simulink model "ASDrf_SelectParameter"  (R2016b)
settings: configuration reference "CodeGenConfigSet" (kept outside this file)
values from neighbouring files (symbols this model uses):
  ASDrf_facGovNegGear0_CUR = Calibration.Parameter    [init_ASDrf_SelectParameter.m]    (also in init_ASDrf_SelectParameter_SIL.m = Simulink.Parameter)
  ASDrf_facGovNegGear0_CURX = Calibration.Parameter    [init_ASDrf_SelectParameter.m]    (also in init_ASDrf_SelectParameter_SIL.m = Simulink.Parameter)
  ASDrf_facGovNegGear1_CUR = Calibration.Parameter    [init_ASDrf_SelectParameter.m]    (also in init_ASDrf_SelectParameter_SIL.m = Simulink.Parameter)
  ASDrf_facGovNegGear1_CURX = Calibration.Parameter    [init_ASDrf_SelectParameter.m]    (also in init_ASDrf_SelectParameter_SIL.m = Simulink.Parameter)
  ASDrf_facGovNegGear2_CUR = Calibration.Parameter    [init_ASDrf_SelectParameter.m]    (also in init_ASDrf_SelectParameter_SIL.m = Simulink.Parameter)
  ASDrf_facGovNegGear2_CURX = Calibration.Parameter    [init_ASDrf_SelectParameter.m]    (also in init_ASDrf_SelectParameter_SIL.m = Simulink.Parameter)
  ASDrf_facGovNegGear3_CUR = Calibration.Parameter    [init_ASDrf_SelectParameter.m]    (also in init_ASDrf_SelectParameter_SIL.m = Simulink.Parameter)
  ASDrf_facGovNegGear3_CURX = Calibration.Parameter    [init_ASDrf_SelectParameter.m]    (also in init_ASDrf_SelectParameter_SIL.m = Simulink.Parameter)
  ASDrf_facGovNegGear4_CUR = Calibration.Parameter    [init_ASDrf_SelectParameter.m]    (also in init_ASDrf_SelectParameter_SIL.m = Simulink.Parameter)
  ASDrf_facGovNegGear4_CURX = Calibration.Parameter    [init_ASDrf_SelectParameter.m]    (also in init_ASDrf_SelectParameter_SIL.m = Simulink.Parameter)
  ASDrf_facGovNegGear5_CUR = Calibration.Parameter    [init_ASDrf_SelectParameter.m]    (also in init_ASDrf_SelectParameter_SIL.m = Simulink.Parameter)
  ASDrf_facGovNegGear5_CURX = Calibration.Parameter    [init_ASDrf_SelectParameter.m]    (also in init_ASDrf_SelectParameter_SIL.m = Simulink.Parameter)
  ASDrf_facGovPosGear0_CUR = Calibration.Parameter    [init_ASDrf_SelectParameter.m]    (also in init_ASDrf_SelectParameter_SIL.m = Simulink.Parameter)
  ASDrf_facGovPosGear0_CURX = Calibration.Parameter    [init_ASDrf_SelectParameter.m]    (also in init_ASDrf_SelectParameter_SIL.m = Simulink.Parameter)
  ASDrf_facGovPosGear1_CUR = Calibration.Parameter    [init_ASDrf_SelectParameter.m]    (also in init_ASDrf_SelectParameter_SIL.m = Simulink.Parameter)
  ASDrf_facGovPosGear1_CURX = Calibration.Parameter    [init_ASDrf_SelectParameter.m]    (also in init_ASDrf_SelectParameter_SIL.m = Simulink.Parameter)
  ASDrf_facGovPosGear2_CUR = Calibration.Parameter    [init_ASDrf_SelectParameter.m]    (also in init_ASDrf_SelectParameter_SIL.m = Simulink.Parameter)
  ASDrf_facGovPosGear2_CURX = Calibration.Parameter    [init_ASDrf_SelectParameter.m]    (also in init_ASDrf_SelectParameter_SIL.m = Simulink.Parameter)
  ASDrf_facGovPosGear3_CUR = Calibration.Parameter    [init_ASDrf_SelectParameter.m]    (also in init_ASDrf_SelectParameter_SIL.m = Simulink.Parameter)
  ASDrf_facGovPosGear3_CURX = Calibration.Parameter    [init_ASDrf_SelectParameter.m]    (also in init_ASDrf_SelectParameter_SIL.m = Simulink.Parameter)
  ASDrf_facGovPosGear4_CUR = Calibration.Parameter    [init_ASDrf_SelectParameter.m]    (also in init_ASDrf_SelectParameter_SIL.m = Simulink.Parameter)
  ASDrf_facGovPosGear4_CURX = Calibration.Parameter    [init_ASDrf_SelectParameter.m]    (also in init_ASDrf_SelectParameter_SIL.m = Simulink.Parameter)
  ASDrf_facGovPosGear5_CUR = Calibration.Parameter    [init_ASDrf_SelectParameter.m]    (also in init_ASDrf_SelectParameter_SIL.m = Simulink.Parameter)
  ASDrf_facGovPosGear5_CURX = Calibration.Parameter    [init_ASDrf_SelectParameter.m]    (also in init_ASDrf_SelectParameter_SIL.m = Simulink.Parameter)
undefined symbols (not defined in the file or in its folder): CEngDsT_tTransf_CURX
settings Model: Creator=lenovo  LastModifiedBy=wangrui
settings ConfigSetRef: SourceLocation=Base Workspace

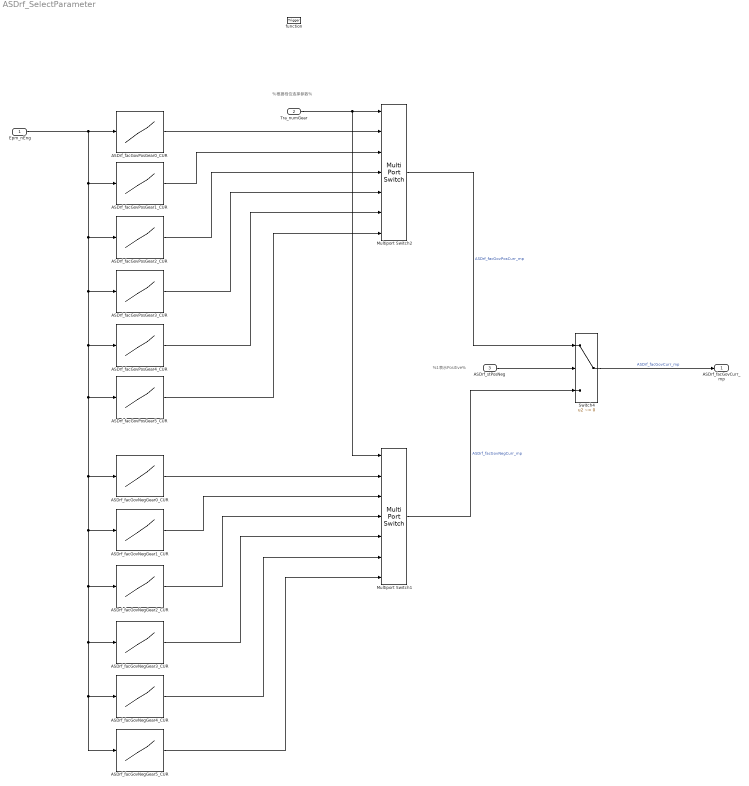
== system ASDrf_SelectParameter ==
  note: %根据档位选择参数%
  note: %1表示Positive%
  Epm_nEng : Inport  Tag=rpm  Description=Engine speed  OutMin=0  OutMax=6000  OutDataTypeStr=EngSpeed_rpm
  Tra_numGear : Inport  Description=Current gear information  Port=2  OutMin=-128  OutMax=127  OutDataTypeStr=Tra_num
  ASDrf_stPosNeg : Inport  Description=Positive or negative intervention status  Port=3  OutMin=0  OutMax=1  OutDataTypeStr=boolean
  function : TriggerPort  TriggerType=function-call  VariantControl=Variant
  ASDrf_facGovNegGear0_CUR : Lookup_n-D  RequirementInfo={} %GIDa_dec7f9a6_086f_4cd9_b948_1532d9a6f0c6  DialogController=Simulink.DDGSource  NumberOfTableDimensions=1  BreakpointsForDimension1=ASDrf_facGovNegGear0_CURX  BreakpointsForDimension2=CEngDsT_tTransf_CURX  IndexSearchMethod=Linear search  BeginIndexSearchUsingPreviousIndexResult=on  Table=ASDrf_facGovNegGear0_CUR  ExtrapMethod=Clip  UseLastTableValue=on  InternalRulePriority=Speed  OutDataTypeStr=Inherit: Inherit via back propagation  SaturateOnIntegerOverflow=on
  ASDrf_facGovNegGear1_CUR : Lookup_n-D  RequirementInfo={} %GIDa_8af62142_568a_4d65_a569_7be54cadb9a5  DialogController=Simulink.DDGSource  NumberOfTableDimensions=1  BreakpointsForDimension1=ASDrf_facGovNegGear1_CURX  BreakpointsForDimension2=CEngDsT_tTransf_CURX  IndexSearchMethod=Linear search  BeginIndexSearchUsingPreviousIndexResult=on  Table=ASDrf_facGovNegGear1_CUR  ExtrapMethod=Clip  UseLastTableValue=on  InternalRulePriority=Speed  OutDataTypeStr=Inherit: Inherit via back propagation  SaturateOnIntegerOverflow=on
  ASDrf_facGovNegGear2_CUR : Lookup_n-D  RequirementInfo={} %GIDa_3d8b842d_bc8c_4451_b7a4_3a6bb0e5109c  DialogController=Simulink.DDGSource  NumberOfTableDimensions=1  BreakpointsForDimension1=ASDrf_facGovNegGear2_CURX  BreakpointsForDimension2=CEngDsT_tTransf_CURX  IndexSearchMethod=Linear search  BeginIndexSearchUsingPreviousIndexResult=on  Table=ASDrf_facGovNegGear2_CUR  ExtrapMethod=Clip  UseLastTableValue=on  InternalRulePriority=Speed  OutDataTypeStr=Inherit: Inherit via back propagation  SaturateOnIntegerOverflow=on
  ASDrf_facGovNegGear3_CUR : Lookup_n-D  RequirementInfo={} %GIDa_717010b1_d4d2_4a42_82df_177817b4661e  DialogController=Simulink.DDGSource  NumberOfTableDimensions=1  BreakpointsForDimension1=ASDrf_facGovNegGear3_CURX  BreakpointsForDimension2=CEngDsT_tTransf_CURX  IndexSearchMethod=Linear search  BeginIndexSearchUsingPreviousIndexResult=on  Table=ASDrf_facGovNegGear3_CUR  ExtrapMethod=Clip  UseLastTableValue=on  InternalRulePriority=Speed  OutDataTypeStr=Inherit: Inherit via back propagation  SaturateOnIntegerOverflow=on
  ASDrf_facGovNegGear4_CUR : Lookup_n-D  RequirementInfo={} %GIDa_d036bcad_9456_44a3_9c9b_0a91d5bad276  DialogController=Simulink.DDGSource  NumberOfTableDimensions=1  BreakpointsForDimension1=ASDrf_facGovNegGear4_CURX  BreakpointsForDimension2=CEngDsT_tTransf_CURX  IndexSearchMethod=Linear search  BeginIndexSearchUsingPreviousIndexResult=on  Table=ASDrf_facGovNegGear4_CUR  ExtrapMethod=Clip  UseLastTableValue=on  InternalRulePriority=Speed  OutDataTypeStr=Inherit: Inherit via back propagation  SaturateOnIntegerOverflow=on
  ASDrf_facGovNegGear5_CUR : Lookup_n-D  RequirementInfo={} %GIDa_4000072d_4691_40fc_9f92_4870488ce3c3  DialogController=Simulink.DDGSource  NumberOfTableDimensions=1  BreakpointsForDimension1=ASDrf_facGovNegGear5_CURX  BreakpointsForDimension2=CEngDsT_tTransf_CURX  IndexSearchMethod=Linear search  BeginIndexSearchUsingPreviousIndexResult=on  Table=ASDrf_facGovNegGear5_CUR  ExtrapMethod=Clip  UseLastTableValue=on  InternalRulePriority=Speed  OutDataTypeStr=Inherit: Inherit via back propagation  SaturateOnIntegerOverflow=on
  ASDrf_facGovPosGear0_CUR : Lookup_n-D  RequirementInfo={} %GIDa_eeb92d19_298b_4c07_9784_ff936e4a1230  DialogController=Simulink.DDGSource  NumberOfTableDimensions=1  BreakpointsForDimension1=ASDrf_facGovPosGear0_CURX  BreakpointsForDimension2=CEngDsT_tTransf_CURX  IndexSearchMethod=Linear search  BeginIndexSearchUsingPreviousIndexResult=on  Table=ASDrf_facGovPosGear0_CUR  ExtrapMethod=Clip  UseLastTableValue=on  InternalRulePriority=Speed  OutDataTypeStr=Inherit: Inherit via back propagation  SaturateOnIntegerOverflow=on
  ASDrf_facGovPosGear1_CUR : Lookup_n-D  RequirementInfo={} %GIDa_79029529_552c_44e4_8a70_6bb176c943a6  DialogController=Simulink.DDGSource  NumberOfTableDimensions=1  BreakpointsForDimension1=ASDrf_facGovPosGear1_CURX  BreakpointsForDimension2=CEngDsT_tTransf_CURX  IndexSearchMethod=Linear search  BeginIndexSearchUsingPreviousIndexResult=on  Table=ASDrf_facGovPosGear1_CUR  ExtrapMethod=Clip  UseLastTableValue=on  InternalRulePriority=Speed  OutDataTypeStr=Inherit: Inherit via back propagation  SaturateOnIntegerOverflow=on
  ASDrf_facGovPosGear2_CUR : Lookup_n-D  RequirementInfo={} %GIDa_3d06e660_b63b_43d5_b51f_660bdd9b60b2  DialogController=Simulink.DDGSource  NumberOfTableDimensions=1  BreakpointsForDimension1=ASDrf_facGovPosGear2_CURX  BreakpointsForDimension2=CEngDsT_tTransf_CURX  IndexSearchMethod=Linear search  BeginIndexSearchUsingPreviousIndexResult=on  Table=ASDrf_facGovPosGear2_CUR  ExtrapMethod=Clip  UseLastTableValue=on  InternalRulePriority=Speed  OutDataTypeStr=Inherit: Inherit via back propagation  SaturateOnIntegerOverflow=on
  ASDrf_facGovPosGear3_CUR : Lookup_n-D  RequirementInfo={} %GIDa_abbb0668_d2b6_4c9e_9b0d_8a1b7749d71a  DialogController=Simulink.DDGSource  NumberOfTableDimensions=1  BreakpointsForDimension1=ASDrf_facGovPosGear3_CURX  BreakpointsForDimension2=CEngDsT_tTransf_CURX  IndexSearchMethod=Linear search  BeginIndexSearchUsingPreviousIndexResult=on  Table=ASDrf_facGovPosGear3_CUR  ExtrapMethod=Clip  UseLastTableValue=on  InternalRulePriority=Speed  OutDataTypeStr=Inherit: Inherit via back propagation  SaturateOnIntegerOverflow=on
  ASDrf_facGovPosGear4_CUR : Lookup_n-D  RequirementInfo={} %GIDa_eb975900_efbf_4ffc_a503_29e29826f2bc  DialogController=Simulink.DDGSource  NumberOfTableDimensions=1  BreakpointsForDimension1=ASDrf_facGovPosGear4_CURX  BreakpointsForDimension2=CEngDsT_tTransf_CURX  IndexSearchMethod=Linear search  BeginIndexSearchUsingPreviousIndexResult=on  Table=ASDrf_facGovPosGear4_CUR  ExtrapMethod=Clip  UseLastTableValue=on  InternalRulePriority=Speed  OutDataTypeStr=Inherit: Inherit via back propagation  SaturateOnIntegerOverflow=on
  ASDrf_facGovPosGear5_CUR : Lookup_n-D  RequirementInfo={} %GIDa_9f826768_612e_48dd_99bc_dcb10a53066c  DialogController=Simulink.DDGSource  NumberOfTableDimensions=1  BreakpointsForDimension1=ASDrf_facGovPosGear5_CURX  BreakpointsForDimension2=CEngDsT_tTransf_CURX  IndexSearchMethod=Linear search  BeginIndexSearchUsingPreviousIndexResult=on  Table=ASDrf_facGovPosGear5_CUR  ExtrapMethod=Clip  UseLastTableValue=on  InternalRulePriority=Speed  OutDataTypeStr=Inherit: Inherit via back propagation  SaturateOnIntegerOverflow=on
  Multiport Switch1 : MultiPortSwitch  DataPortOrder=Zero-based contiguous  Inputs=6  DataPortIndices={5,4,3,2,1,0}
  Multiport Switch2 : MultiPortSwitch  DataPortOrder=Zero-based contiguous  Inputs=6  DataPortIndices={5,4,3,2,1,0}
  Switch4 : Switch  Criteria=u2 ~= 0  SaturateOnIntegerOverflow=on  InputSameDT=on
  ASDrf_facGovCurr_mp : Outport  Description=Active state after priorisation (decimal coded)  OutMin=0  OutMax=99.9  OutDataTypeStr=PT_fac
  wires:
  Switch4/1 -> ASDrf_facGovCurr_mp/1  "ASDrf_facGovCurr_mp"
  ASDrf_stPosNeg/1 -> Switch4/2
  Multiport Switch2/1 -> Switch4/1  "ASDrf_facGovPosCurr_mp"
  Multiport Switch1/1 -> Switch4/3  "ASDrf_facGovNegCurr_mp"
  Tra_numGear/1 -> Multiport Switch2/1, Multiport Switch1/1
  Epm_nEng/1 -> ASDrf_facGovPosGear0_CUR/1, ASDrf_facGovPosGear1_CUR/1, ASDrf_facGovPosGear2_CUR/1, ASDrf_facGovPosGear3_CUR/1, ASDrf_facGovPosGear4_CUR/1, ASDrf_facGovPosGear5_CUR/1, ASDrf_facGovNegGear0_CUR/1, ASDrf_facGovNegGear1_CUR/1, ASDrf_facGovNegGear2_CUR/1, ASDrf_facGovNegGear3_CUR/1, ASDrf_facGovNegGear4_CUR/1, ASDrf_facGovNegGear5_CUR/1
  ASDrf_facGovPosGear0_CUR/1 -> Multiport Switch2/2
  ASDrf_facGovPosGear1_CUR/1 -> Multiport Switch2/3
  ASDrf_facGovPosGear2_CUR/1 -> Multiport Switch2/4
  ASDrf_facGovPosGear3_CUR/1 -> Multiport Switch2/5
  ASDrf_facGovPosGear4_CUR/1 -> Multiport Switch2/6
  ASDrf_facGovPosGear5_CUR/1 -> Multiport Switch2/7
  ASDrf_facGovNegGear0_CUR/1 -> Multiport Switch1/2
  ASDrf_facGovNegGear1_CUR/1 -> Multiport Switch1/3
  ASDrf_facGovNegGear2_CUR/1 -> Multiport Switch1/4
  ASDrf_facGovNegGear3_CUR/1 -> Multiport Switch1/5
  ASDrf_facGovNegGear4_CUR/1 -> Multiport Switch1/6
  ASDrf_facGovNegGear5_CUR/1 -> Multiport Switch1/7
